simulink subsystem "lstm_turboShaftEngine"  (R2023a)
settings: Solver=VariableStepAuto  StartTime=0.0  StopTime=10.0  RelTol=1e-3
undefined symbols (not defined in the file): rom
libraries: deeplib x1
settings Model: Creator=imyrsini  LastModifiedBy=imyrsini

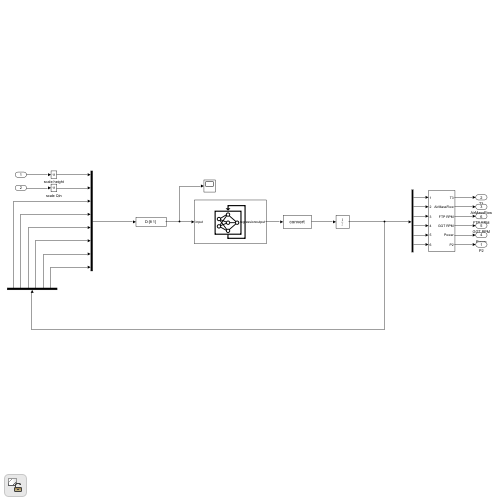
[thumbnail: Simulink's stored preview of the top-level diagram]
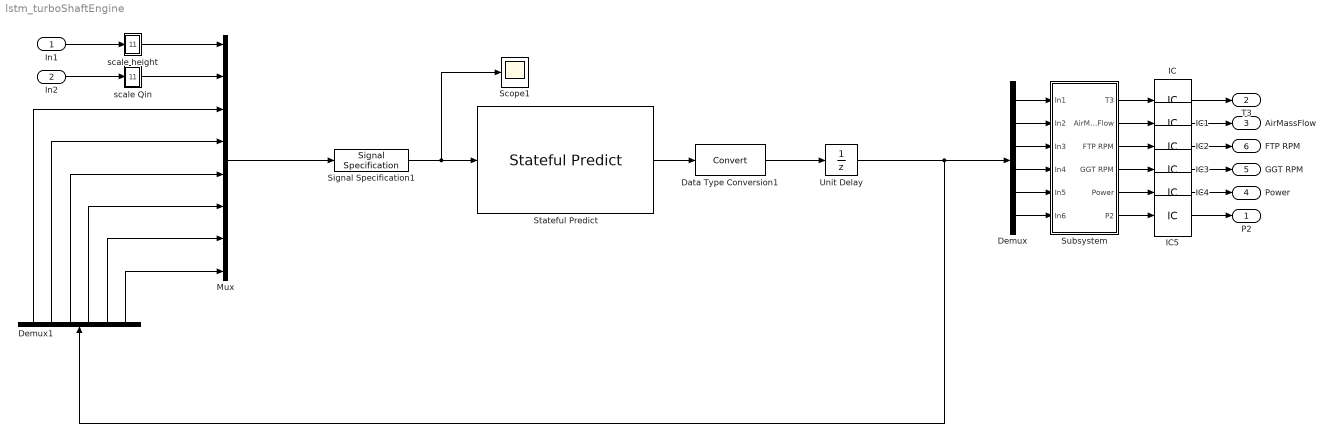
== system lstm_turboShaftEngine ==
  In1 : Inport
  In2 : Inport  Port=2
  Data Type Conversion1 : DataTypeConversion  SaturateOnIntegerOverflow=off  RndMeth=Floor
  Demux : Demux  Outputs=6
  Demux1 : Demux  Outputs=6
  IC : InitialCondition  Value=1000
  IC1 : InitialCondition  Value=5
  IC2 : InitialCondition  Value=2e4
  IC3 : InitialCondition  Value=3e4
  IC4 : InitialCondition  Value=2e3
  IC5 : InitialCondition  Value=1e5
  Mux : Mux  Inputs=8
  Scope1 : Scope
  Signal Specification1 : SignalSpecification  Dimensions=[8 1]
  Stateful Predict : deeplib/Stateful Predict  Network=Network from MAT-file  NetworkFunction=untitled  NetworkFilePath=C:\Users\imyrsini\OneDrive - MathWorks\Documents\Projects\AEprojects\LSTM Model Reduction\turboshaftEngine_ROM\turboshaft_ROM.mat  InputDataFormats={'',''}  SampleTime=-1  ForceInterpretedSim=off  EnableDLNetwork=on
  Subsystem : Subsystem
  Unit Delay : UnitDelay  InitialCondition=|  SampleTime=-1  HasFrameUpgradeWarning=on
      | [    0.8831
      | ;    1.5615;
      |     1.1017;
      |     1.0655
      | ;    1.1803;
      |     1.4918]
  scale Qin : Subsystem
  scale height : Subsystem
  P2 : Outport
  T3 : Outport  Port=2
  AirMassFlow : Outport  Port=3
  Power : Outport  Port=4
  GGT RPM : Outport  Port=5
  FTP RPM : Outport  Port=6
  wires:
  Signal Specification1/1 -> Stateful Predict/1, Scope1/1
  Mux/1 -> Signal Specification1/1
  Demux1/6 -> Mux/8
  Stateful Predict/1 -> Data Type Conversion1/1
  Data Type Conversion1/1 -> Unit Delay/1
  Unit Delay/1 -> Demux1/1, Demux/1
  Demux1/1 -> Mux/3
  Demux1/5 -> Mux/7
  Demux1/4 -> Mux/6
  Demux1/3 -> Mux/5
  Demux1/2 -> Mux/4
  In2/1 -> scale Qin/1(In1)
  In1/1 -> scale height/1(In1)
  scale height/1(Out1) -> Mux/1
  scale Qin/1(Out1) -> Mux/2
  Demux/1 -> Subsystem/1(In1)
  Demux/2 -> Subsystem/2(In2)
  Demux/3 -> Subsystem/3(In3)
  Demux/4 -> Subsystem/4(In4)
  Demux/5 -> Subsystem/5(In5)
  Demux/6 -> Subsystem/6(In6)
  Subsystem/1(T3) -> IC/1
  Subsystem/2(AirMassFlow) -> IC1/1
  Subsystem/3(FTP RPM) -> IC2/1
  Subsystem/4(GGT RPM) -> IC3/1
  Subsystem/5(Power) -> IC4/1
  Subsystem/6(P2) -> IC5/1
  IC/1 -> T3/1
  IC1/1 -> AirMassFlow/1
  IC2/1 -> FTP RPM/1
  IC3/1 -> GGT RPM/1
  IC4/1 -> Power/1
  IC5/1 -> P2/1

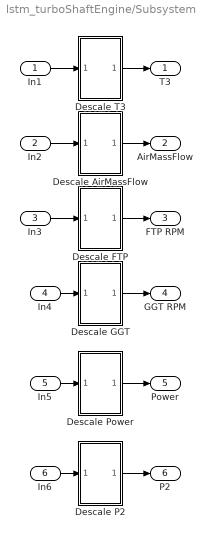
== system lstm_turboShaftEngine/Subsystem ==
  In1 : Inport
  In2 : Inport  Port=2
  In3 : Inport  Port=3
  In4 : Inport  Port=4
  In5 : Inport  Port=5
  In6 : Inport  Port=6
  Descale AirMassFlow : Subsystem
  Descale FTP : Subsystem
  Descale GGT : Subsystem
  Descale P2 : Subsystem
  Descale Power : Subsystem
  Descale T3 : Subsystem
  T3 : Outport
  AirMassFlow : Outport  Port=2
  FTP RPM : Outport  Port=3
  GGT RPM : Outport  Port=4
  Power : Outport  Port=5
  P2 : Outport  Port=6
  wires:
  Descale P2/1(Out1) -> P2/1
  In6/1 -> Descale P2/1(In1)
  In5/1 -> Descale Power/1(In1)
  In4/1 -> Descale GGT/1(In1)
  Descale T3/1(Out1) -> T3/1
  In2/1 -> Descale AirMassFlow/1(In1)
  In3/1 -> Descale FTP/1(In1)
  In1/1 -> Descale T3/1(In1)
  Descale Power/1(Out1) -> Power/1
  Descale FTP/1(Out1) -> FTP RPM/1
  Descale AirMassFlow/1(Out1) -> AirMassFlow/1
  Descale GGT/1(Out1) -> GGT RPM/1

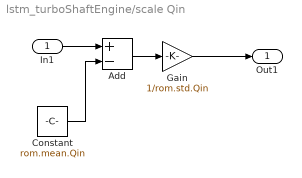
== system lstm_turboShaftEngine/scale Qin ==
  In1 : Inport
  Add : Sum  Inputs=+-
  Constant : Constant  Value=rom.mean.Qin
  Gain : Gain  Gain=1/rom.std.Qin
  Out1 : Outport
  wires:
  In1/1 -> Add/1
  Constant/1 -> Add/2
  Add/1 -> Gain/1
  Gain/1 -> Out1/1

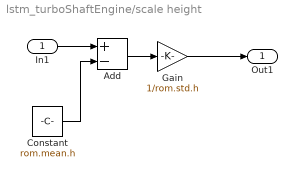
== system lstm_turboShaftEngine/scale height ==
  In1 : Inport
  Add : Sum  Inputs=+-
  Constant : Constant  Value=rom.mean.h
  Gain : Gain  Gain=1/rom.std.h
  Out1 : Outport
  wires:
  Gain/1 -> Out1/1
  Add/1 -> Gain/1
  Constant/1 -> Add/2
  In1/1 -> Add/1

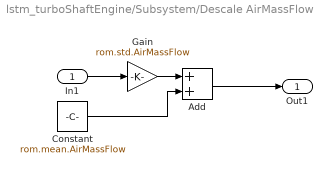
== system lstm_turboShaftEngine/Subsystem/Descale AirMassFlow ==
  In1 : Inport
  Add : Sum
  Constant : Constant  Value=rom.mean.AirMassFlow
  Gain : Gain  Gain=rom.std.AirMassFlow
  Out1 : Outport
  wires:
  In1/1 -> Gain/1
  Add/1 -> Out1/1
  Gain/1 -> Add/1
  Constant/1 -> Add/2

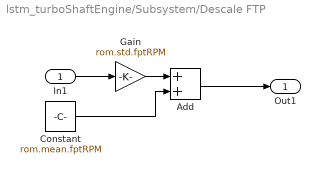
== system lstm_turboShaftEngine/Subsystem/Descale FTP ==
  In1 : Inport
  Add : Sum
  Constant : Constant  Value=rom.mean.fptRPM
  Gain : Gain  Gain=rom.std.fptRPM
  Out1 : Outport
  wires:
  Constant/1 -> Add/2
  Gain/1 -> Add/1
  Add/1 -> Out1/1
  In1/1 -> Gain/1

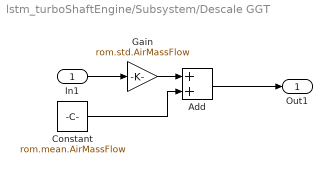
== system lstm_turboShaftEngine/Subsystem/Descale GGT ==
  In1 : Inport
  Add : Sum
  Constant : Constant  Value=rom.mean.AirMassFlow
  Gain : Gain  Gain=rom.std.AirMassFlow
  Out1 : Outport
  wires:
  In1/1 -> Gain/1
  Add/1 -> Out1/1
  Gain/1 -> Add/1
  Constant/1 -> Add/2

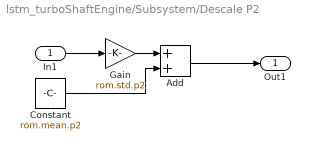
== system lstm_turboShaftEngine/Subsystem/Descale P2 ==
  In1 : Inport
  Add : Sum
  Constant : Constant  Value=rom.mean.p2
  Gain : Gain  Gain=rom.std.p2
  Out1 : Outport
  wires:
  In1/1 -> Gain/1
  Add/1 -> Out1/1
  Gain/1 -> Add/1
  Constant/1 -> Add/2

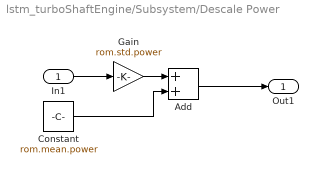
== system lstm_turboShaftEngine/Subsystem/Descale Power ==
  In1 : Inport
  Add : Sum
  Constant : Constant  Value=rom.mean.power
  Gain : Gain  Gain=rom.std.power
  Out1 : Outport
  wires:
  Constant/1 -> Add/2
  Gain/1 -> Add/1
  Add/1 -> Out1/1
  In1/1 -> Gain/1

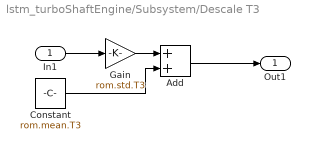
== system lstm_turboShaftEngine/Subsystem/Descale T3 ==
  In1 : Inport
  Add : Sum
  Constant : Constant  Value=rom.mean.T3
  Gain : Gain  Gain=rom.std.T3
  Out1 : Outport
  wires:
  Constant/1 -> Add/2
  Gain/1 -> Add/1
  Add/1 -> Out1/1
  In1/1 -> Gain/1
